simulink model "OL_VC"  (R2022b)
settings: Solver=VariableStepAuto  StartTime=0.0  StopTime=10.0  RelTol=1e-3
settings Model: Creator=marcu  LastModifiedBy=marcu

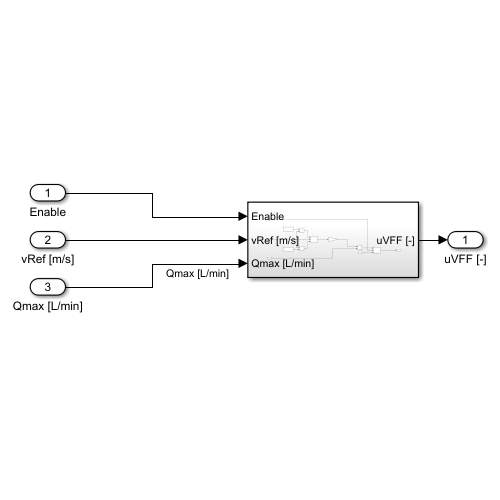
[thumbnail: Simulink's stored preview of the top-level diagram]
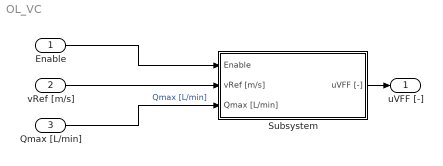
== system OL_VC ==
  Enable : Inport
  vRef [m/s] : Inport  Port=2
  Qmax [L/min] : Inport  Port=3
  Subsystem : Subsystem
  uVFF [-] : Outport
  wires:
  Enable/1 -> Subsystem/1(Enable)
  vRef [m/s]/1 -> Subsystem/2(vRef [m/s])
  Qmax [L/min]/1 -> Subsystem/3(Qmax [L/min])  "Qmax [L/min]"
  Subsystem/1(uVFF [-]) -> uVFF [-]/1

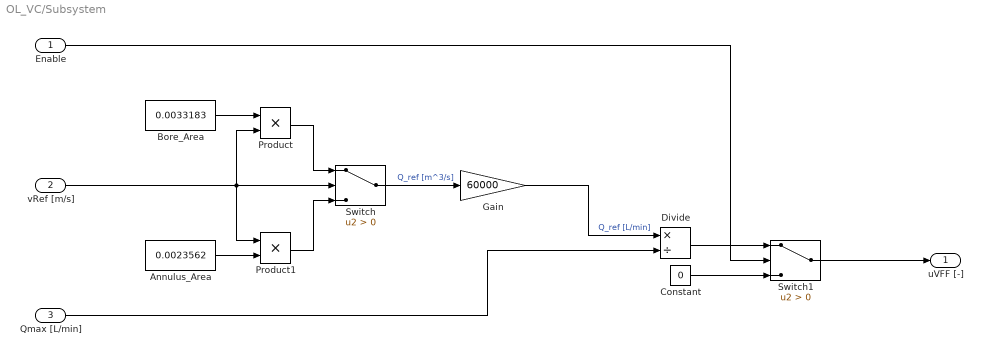
== system OL_VC/Subsystem ==
  Enable : Inport
  vRef [m/s] : Inport  Port=2
  Qmax [L/min] : Inport  Port=3
  Annulus_Area : Constant  Value=0.0023562
  Bore_Area : Constant  Value=0.0033183
  Constant : Constant  Value=0
  Divide : Product  Inputs=*/
  Gain : Gain  Gain=60000
  Product : Product
  Product1 : Product
  Switch : Switch  Criteria=u2 > Threshold  SaturateOnIntegerOverflow=off  InputSameDT=off
  Switch1 : Switch  Criteria=u2 > Threshold  SaturateOnIntegerOverflow=off  InputSameDT=off
  uVFF [-] : Outport
  wires:
  vRef [m/s]/1 -> Product/2, Product1/1, Switch/2
  Qmax [L/min]/1 -> Divide/2
  Gain/1 -> Divide/1  "Q_ref [L/min]"
  Product/1 -> Switch/1
  Divide/1 -> Switch1/1
  Switch/1 -> Gain/1  "Q_ref [m^3/s]"
  Constant/1 -> Switch1/3
  Bore_Area/1 -> Product/1
  Product1/1 -> Switch/3
  Enable/1 -> Switch1/2
  Annulus_Area/1 -> Product1/2
  Switch1/1 -> uVFF [-]/1
